simulink library "TimeSharedLib"  (R2023a)
settings: Solver=VariableStepAuto  StartTime=0.0  StopTime=10.0  RelTol=1e-3
libraries: NSA_DEVS_LOGISTICS_ATOMIC x10, NSA_DEVS_STATISTICS_ATOMIC x1, NSA_DEVS_ROUTING_ATOMIC x1, NSA_DEVS_LOGISTICS_COUPLED x1, NSA_DEVS_MATH_OPERATIONS_ATOMIC x1, NSA_DEVS_SOURCES_ATOMIC x1
settings Model: Creator=peter  LastModifiedBy=peter

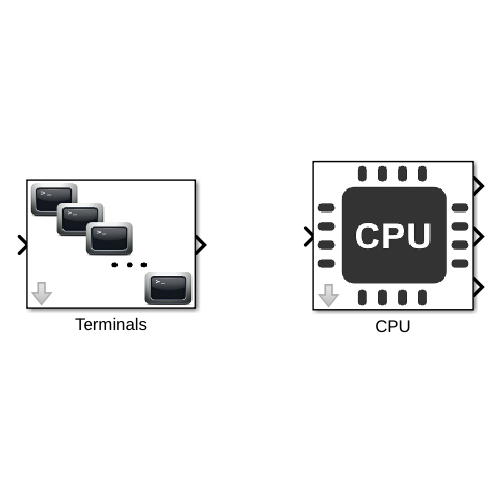
[thumbnail: Simulink's stored preview of the top-level diagram]
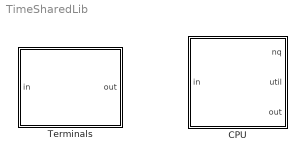
== system TimeSharedLib ==
  CPU : Subsystem  mask{q=0.1, tSwap=0.01}
      mask prompts: q "Time slice"; tSwap "Swap time"
      mask Display: image('$imagefile'); % Use "Edit Image" on toolstrip to change.
  Terminals : Subsystem  mask{N=3, tW=1, tS=1}
      mask prompts: N "Number of terminals"; tW "Waiting time"; tS "Service time"
      mask Display: image('$imagefile'); % Use "Edit Image" on toolstrip to change.

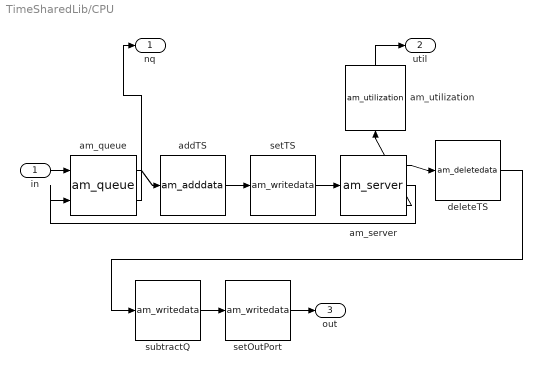
== system TimeSharedLib/CPU ==
  in : Inport
  addTS : NSA_DEVS_LOGISTICS_ATOMIC/am_adddata  fields="[\"tSlice\"]"  values="[\"1\"]"  numeric=[true]  infield="\"id\""  tau=[0,0.25]  debug=0
      settings: SourceProductName=NSA_DEVS
  am_queue : NSA_DEVS_LOGISTICS_ATOMIC/am_queue  tD=[0,2]  tau=[0,1]  debug=0
      settings: SourceProductName=NSA_DEVS
  am_server : NSA_DEVS_LOGISTICS_ATOMIC/am_server  tS=1.0  tsField="\"tSlice\""  tau=[0,1]  debug=0
      settings: SourceProductName=NSA_DEVS
  am_utilization : NSA_DEVS_STATISTICS_ATOMIC/am_utilization  tau=[0,1]  debug=0
      settings: SourceProductName=NSA_DEVS
  deleteTS : NSA_DEVS_LOGISTICS_ATOMIC/am_deletedata  fields="\"tSlice\""  tau=[0,0.25]  debug=0
      settings: SourceProductName=NSA_DEVS
  setOutPort : NSA_DEVS_LOGISTICS_ATOMIC/am_writedata  inFields="[\"remainingServiceTime\"]"  outField="\"outPort\""  changeFunc="\"out = 1 + (in(1) > 0);\""  tau=[0,0.25]  debug=0
      settings: SourceProductName=NSA_DEVS
  setTS : NSA_DEVS_LOGISTICS_ATOMIC/am_writedata  inFields="[\"remainingServiceTime\"]"  outField="\"tSlice\""  changeFunc="\"out = min(\" + q + \", in(1)) + \" + tSwap + \";\""  tau=[0,0.25]  debug=0
      settings: SourceProductName=NSA_DEVS
  subtractQ : NSA_DEVS_LOGISTICS_ATOMIC/am_writedata  inFields="[\"remainingServiceTime\"]"  outField="\"remainingServiceTime\""  changeFunc="\"out = max(in(1) - \" + q + \", 0);\""  tau=[0,0.25]  debug=0
      settings: SourceProductName=NSA_DEVS
  nq : Outport
  util : Outport  Port=2
  out : Outport  Port=3
  wires:
  in/1 -> am_queue/1
  am_server/1 -> deleteTS/1
  am_queue/2 -> nq/1
  am_server/2 -> am_queue/2
  setTS/1 -> am_server/1
  am_queue/1 -> addTS/1
  addTS/1 -> setTS/1
  deleteTS/1 -> subtractQ/1
  subtractQ/1 -> setOutPort/1
  setOutPort/1 -> out/1
  am_server/3 -> am_utilization/1
  am_utilization/1 -> util/1

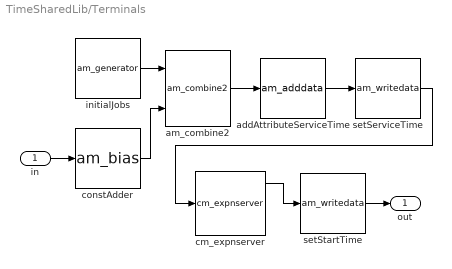
== system TimeSharedLib/Terminals ==
  in : Inport
  addAttributeServiceTime : NSA_DEVS_LOGISTICS_ATOMIC/am_adddata  fields="[\"remainingServiceTime\", \"outPort\", \"startTime\"]"  values=[0, 1, 0]  numeric=[true, true, true]  infield="\"id\""  tau=[0,1]  debug=0
      settings: SourceProductName=NSA_DEVS
  am_combine2 : NSA_DEVS_ROUTING_ATOMIC/am_combine2  tD=[0,2]  tau=[0,1]  debug=0
      settings: SourceProductName=NSA_DEVS
  cm_expnserver : NSA_DEVS_LOGISTICS_COUPLED/cm_expnserver  N=N  tS=tW  fieldname="\"waitingTime\""  tau=[0,1]  debug=0
      settings: SourceProductName=NSA_DEVS
  constAdder : NSA_DEVS_MATH_OPERATIONS_ATOMIC/am_bias  bias=N  tau=[0,1]  debug=0
      settings: SourceProductName=NSA_DEVS
  initialJobs : NSA_DEVS_SOURCES_ATOMIC/am_generator  tG=0  n0=1  nG=N  tD=[0,2]  debug=0
      settings: SourceProductName=NSA_DEVS
  setServiceTime : NSA_DEVS_LOGISTICS_ATOMIC/am_writedata  inFields=[]  outField="\"remainingServiceTime\""  changeFunc="\"out = -\" + tS + \"*log(rand());\""  tau=[0,1]  debug=0
      settings: SourceProductName=NSA_DEVS
  setStartTime : NSA_DEVS_LOGISTICS_ATOMIC/am_writedata  inFields=[]  outField="\"startTime\""  changeFunc="\"out = get_time();\""  tau=[0,1]  debug=0
      settings: SourceProductName=NSA_DEVS
  out : Outport
  wires:
  initialJobs/1 -> am_combine2/1
  am_combine2/1 -> addAttributeServiceTime/1
  addAttributeServiceTime/1 -> setServiceTime/1
  in/1 -> constAdder/1
  constAdder/1 -> am_combine2/2
  setServiceTime/1 -> cm_expnserver/1
  cm_expnserver/1 -> setStartTime/1
  setStartTime/1 -> out/1
